simulink model "Quad_Nonlinear_LQDG"  (R2020a)
settings: Solver=ode4  StartTime=0.0  StopTime=1  FixedStep=0.02  RelTol=1e-3
InitFcn:
  | init
undefined symbols (not defined in the file or in its folder): A1, A2, A3, A4, A5, B1, B2, B3, B4, B5, C1, C2, C3, magnitude, rad, s, weighting_matrix, x0
libraries: aerolibconvert2 x4
settings Model: Creator=Ali  LastModifiedBy=Ali
settings SolverCC: AlgebraicLoopSolver=LineSearch

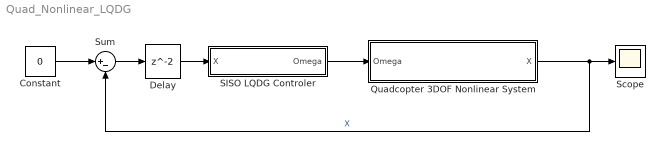
== system Quad_Nonlinear_LQDG ==
  Constant : Constant  Value=0
  Delay : Delay
  Quadcopter 3DOF Nonlinear System : Subsystem  TreatAsAtomicUnit=on
  SISO LQDG Controler : Subsystem
  Scope : Scope
  Sum : Sum  Inputs=|+-
  wires:
  Quadcopter 3DOF Nonlinear System/1(X) -> Sum/2, Scope/1  "X"
  Sum/1 -> Delay/1
  Constant/1 -> Sum/1
  Delay/1 -> SISO LQDG Controler/1(X)
  SISO LQDG Controler/1(Omega) -> Quadcopter 3DOF Nonlinear System/1(Omega)

== system Quad_Nonlinear_LQDG/Quadcopter 3DOF Nonlinear System ==
  Omega : Inport
  Integrator : Integrator  InitialCondition=x0
  Quad System : Subsystem
  Subsystem : Subsystem
  X : Outport
  wires:
  Integrator/1 -> Quad System/1(X), X/1  "X"
  Quad System/1(dot(X)) -> Integrator/1  "dot(X)"
  Omega/1 -> Subsystem/1(motor command)
  Subsystem/1(motor output) -> Quad System/2(Omega)

== system Quad_Nonlinear_LQDG/SISO LQDG Controler ==
  X : Inport
  Angular Velocity Conversion : aerolibconvert2/Angular Velocity Conversion  IU=rad/s  OU=rpm
  Angular Velocity Conversion1 : aerolibconvert2/Angular Velocity Conversion  IU=rpm  OU=rad/s
  SISO LQDG : Subsystem
  Saturation : Saturate  UpperLimit=6000  LowerLimit=1300
  u2Omega : Subsystem
  Omega : Outport
  wires:
  X/1 -> SISO LQDG/1(X)
  SISO LQDG/1(u) -> u2Omega/1(u)
  Angular Velocity Conversion/1 -> Saturation/1
  Saturation/1 -> Angular Velocity Conversion1/1
  u2Omega/1(Omega) -> Angular Velocity Conversion/1
  Angular Velocity Conversion1/1 -> Omega/1

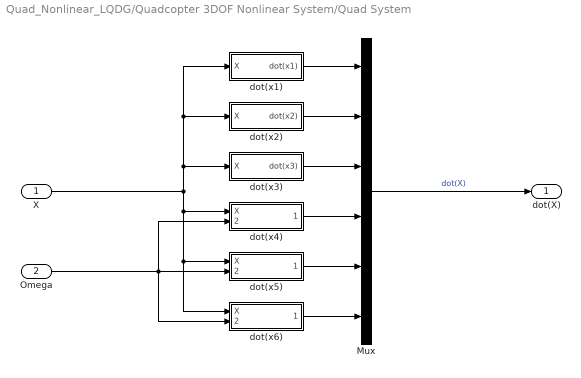
== system Quad_Nonlinear_LQDG/Quadcopter 3DOF Nonlinear System/Quad System ==
  X : Inport
  Omega : Inport  Port=2
  Mux : Mux  Inputs=6
  dot(x1) : Subsystem
  dot(x2) : Subsystem
  dot(x3) : Subsystem
  dot(x4) : Subsystem
  dot(x5) : Subsystem
  dot(x6) : Subsystem
  dot(X) : Outport
  wires:
  Mux/1 -> dot(X)/1  "dot(X)"
  X/1 -> dot(x1)/1(X), dot(x2)/1(X), dot(x3)/1(X), dot(x6)/1(X), dot(x5)/1(X), dot(x4)/1(X)
  Omega/1 -> dot(x4)/2(Omega), dot(x6)/2(Omega), dot(x5)/2(Omega)
  dot(x5)/1(dot(x5)) -> Mux/5
  dot(x2)/1(dot(x2)) -> Mux/2
  dot(x4)/1(dot(x4)) -> Mux/4
  dot(x3)/1(dot(x3)) -> Mux/3
  dot(x1)/1(dot(x1)) -> Mux/1
  dot(x6)/1(dot(x6)) -> Mux/6

== system Quad_Nonlinear_LQDG/Quadcopter 3DOF Nonlinear System/Subsystem ==
  motor command : Inport
  Angular Velocity Conversion : aerolibconvert2/Angular Velocity Conversion  IU=rad/s  OU=rpm
  Angular Velocity Conversion1 : aerolibconvert2/Angular Velocity Conversion  IU=rpm  OU=rad/s
  Mototr Transfer function : Subsystem
  Saturation : Saturate  UpperLimit=6000  LowerLimit=1300
  duty2rpm_Emax1 : Lookup_n-D  NumberOfTableDimensions=1  BreakpointsForDimension1=|  Table=|  RndMeth=Simplest  InputSameDT=on
      BreakpointsForDimension1=|
      | [0.5
      | 0.55
      | 0.6
      | 0.65
      | 0.7
      | 0.75
      | 0.8
      | 0.85
      | 0.9
      | 0.95
      | 1]
      Table=|
      | [1201
      | 2305
      | 3096
      | 3930
      | 4118
      | 4555
      | 5122
      | 5552
      | 5957
      | 6291
      | 6360]
  rpm2duty_Emax : Lookup_n-D  NumberOfTableDimensions=1  BreakpointsForDimension1=|  Table=|  RndMeth=Simplest  InputSameDT=on
      BreakpointsForDimension1=|
      | [1201
      | 2305
      | 3096
      | 3930
      | 4118
      | 4555
      | 5122
      | 5552
      | 5957
      | 6291
      | 6360]
      Table=|
      | [0.5
      | 0.55
      | 0.6
      | 0.65
      | 0.7
      | 0.75
      | 0.8
      | 0.85
      | 0.9
      | 0.95
      | 1]
  motor output : Outport
  wires:
  motor command/1 -> Angular Velocity Conversion/1
  Saturation/1 -> rpm2duty_Emax/1
  Angular Velocity Conversion/1 -> Saturation/1
  duty2rpm_Emax1/1 -> Angular Velocity Conversion1/1
  Angular Velocity Conversion1/1 -> motor output/1
  rpm2duty_Emax/1 -> Mototr Transfer function/1(In1)
  Mototr Transfer function/1(Out1) -> duty2rpm_Emax1/1

== system Quad_Nonlinear_LQDG/SISO LQDG Controler/SISO LQDG ==
  X : Inport
  Mux : Mux  Inputs=3
  Pitch LQDG Controller : Subsystem
  Roll LQDG Controller : Subsystem
  Subsystem : Subsystem
  Yaw LQDG Controller : Subsystem
  u : Outport
  wires:
  Mux/1 -> u/1  "u"
  X/1 -> Subsystem/1(X)
  Subsystem/1(roll) -> Roll LQDG Controller/1(roll)
  Roll LQDG Controller/1(u1) -> Mux/1
  Subsystem/2(pitch) -> Pitch LQDG Controller/1(pitch)
  Pitch LQDG Controller/1(u2) -> Mux/2
  Subsystem/3(yaw) -> Yaw LQDG Controller/1(yaw)
  Yaw LQDG Controller/1(u3) -> Mux/3

== system Quad_Nonlinear_LQDG/SISO LQDG Controler/u2Omega ==
  u : Inport
  MATLAB Function1 : MATLAB Function  TreatAsAtomicUnit=on
  Mux1 : Mux
  Omega : Outport
  wires:
  Mux1/1 -> Omega/1
  MATLAB Function1/2(omega_2) -> Mux1/2
  u/1 -> MATLAB Function1/1(u)
  MATLAB Function1/3(omega_3) -> Mux1/3
  MATLAB Function1/1(omega_1) -> Mux1/1
  MATLAB Function1/4(omega_4) -> Mux1/4

== system Quad_Nonlinear_LQDG/Quadcopter 3DOF Nonlinear System/Quad System/dot(x1) ==
  X : Inport
  1 : Subsystem
  Add : Sum  Inputs=+++
  Subsystem : Subsystem
  Subsystem1 : Subsystem
  dot(x1) : Outport
  wires:
  X/1 -> Subsystem1/1(X), Subsystem/1(X), 1/1(X)  "X"
  Subsystem1/1(x4) -> Add/3
  Subsystem/1(x6cos(x1)tan(x2)) -> Add/2
  Add/1 -> dot(x1)/1
  1/1(x5sin(x1)tan(x2)) -> Add/1

== system Quad_Nonlinear_LQDG/Quadcopter 3DOF Nonlinear System/Quad System/dot(x2) ==
  X : Inport
  1 : Subsystem
  Add : Sum  Inputs=+-
  Subsystem : Subsystem
  dot(x2) : Outport
  wires:
  X/1 -> 1/1(X), Subsystem/1(X)  "X"
  Subsystem/1(x6sin(x1)) -> Add/2
  Add/1 -> dot(x2)/1
  1/1(x5cos(x1)) -> Add/1

== system Quad_Nonlinear_LQDG/Quadcopter 3DOF Nonlinear System/Quad System/dot(x3) ==
  X : Inport
  1 : Subsystem
  Add : Sum
  Product : Product
  Subsystem : Subsystem
  Subsystem1 : Subsystem
  dot(x3) : Outport
  wires:
  X/1 -> Subsystem1/1(X), Subsystem/1(X), 1/1(X)  "X"
  Subsystem/1(x6cos(x1)) -> Add/2
  1/1(x5sin(x1)) -> Add/1
  Product/1 -> dot(x3)/1
  Add/1 -> Product/1
  Subsystem1/1(sec(x2)) -> Product/2

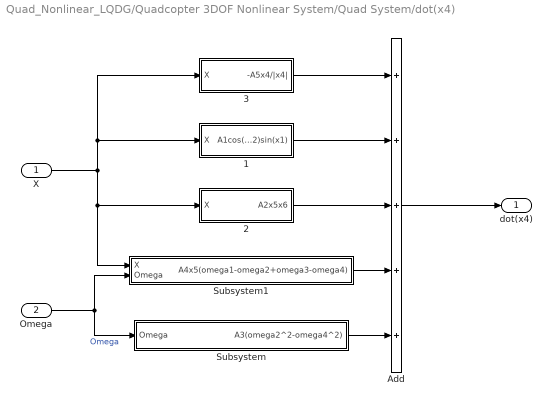
== system Quad_Nonlinear_LQDG/Quadcopter 3DOF Nonlinear System/Quad System/dot(x4) ==
  X : Inport
  Omega : Inport  Port=2
  1 : Subsystem
  2 : Subsystem
  3 : Subsystem
  Add : Sum  Inputs=+++++
  Subsystem : Subsystem
  Subsystem1 : Subsystem
  dot(x4) : Outport
  wires:
  X/1 -> Subsystem1/1(X), 2/1(X), 3/1(X), 1/1(X)
  Omega/1 -> Subsystem1/2(Omega), Subsystem/1(Omega)  "Omega"
  Add/1 -> dot(x4)/1
  3/1("-A5x4/|x4| ") -> Add/1
  1/1(A1cos(x2)sin(x1)) -> Add/2
  2/1(A2x5x6) -> Add/3
  Subsystem1/1(A4x5(omega1-omega2+omega3-omega4)) -> Add/4
  Subsystem/1(A3(omega2^2-omega4^2)) -> Add/5

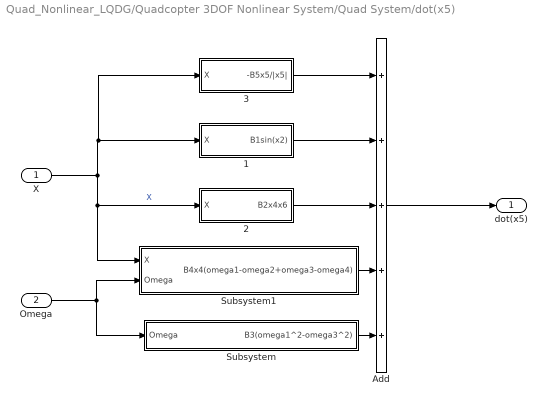
== system Quad_Nonlinear_LQDG/Quadcopter 3DOF Nonlinear System/Quad System/dot(x5) ==
  X : Inport
  Omega : Inport  Port=2
  1 : Subsystem
  2 : Subsystem
  3 : Subsystem
  Add : Sum  Inputs=+++++
  Subsystem : Subsystem
  Subsystem1 : Subsystem
  dot(x5) : Outport
  wires:
  X/1 -> Subsystem1/1(X), 2/1(X), 3/1(X), 1/1(X)  "X"
  Omega/1 -> Subsystem/1(Omega), Subsystem1/2(Omega)
  Add/1 -> dot(x5)/1
  3/1("-B5x5/|x5| ") -> Add/1
  1/1(B1sin(x2)) -> Add/2
  2/1(B2x4x6) -> Add/3
  Subsystem1/1(B4x4(omega1-omega2+omega3-omega4)) -> Add/4
  Subsystem/1(B3(omega1^2-omega3^2)) -> Add/5

== system Quad_Nonlinear_LQDG/Quadcopter 3DOF Nonlinear System/Quad System/dot(x6) ==
  X : Inport
  Omega : Inport  Port=2
  2 : Subsystem
  3 : Subsystem
  Add : Sum  Inputs=+++
  Subsystem : Subsystem
  dot(x6) : Outport
  wires:
  Omega/1 -> Subsystem/1(Omega)  "Omega"
  Add/1 -> dot(x6)/1
  3/1("-C3x6/|x6| ") -> Add/1
  2/1(C1x4x5) -> Add/2
  Subsystem/1(C2(omega1^2-omega2^2+omega3^2-omega4^2)) -> Add/3
  X/1 -> 3/1(X), 2/1(X)  "X"

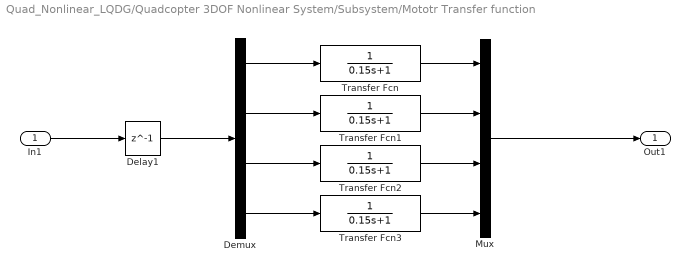
== system Quad_Nonlinear_LQDG/Quadcopter 3DOF Nonlinear System/Subsystem/Mototr Transfer function ==
  In1 : Inport
  Delay1 : Delay  DelayLength=1
  Demux : Demux
  Mux : Mux
  Transfer Fcn{,1..3} (4 alike) : TransferFcn  Denominator=[0.15 1]
  Out1 : Outport
  wires:
  Mux/1 -> Out1/1
  Transfer Fcn/1 -> Mux/1
  Delay1/1 -> Demux/1
  Demux/1 -> Transfer Fcn/1
  Transfer Fcn1/1 -> Mux/2
  Demux/3 -> Transfer Fcn2/1
  In1/1 -> Delay1/1
  Demux/2 -> Transfer Fcn1/1
  Transfer Fcn3/1 -> Mux/4
  Transfer Fcn2/1 -> Mux/3
  Demux/4 -> Transfer Fcn3/1

== system Quad_Nonlinear_LQDG/SISO LQDG Controler/SISO LQDG/Pitch LQDG Controller ==
  pitch : Inport
  Constant : Constant  Value=B1
  Constant1 : Constant  Value=B3
  Demux : Demux  Outputs=3
  Pitch function : MATLAB Function  TreatAsAtomicUnit=on
  Selector : Selector  InputPortWidth=5  IndexOptions=Index vector (dialog)  Indices=[1 3 5]  OutputSizes=1
  weighting matrix for distubance and noise using TCACS : Constant  Value=weighting_matrix
  u2 : Outport
  wires:
  Pitch function/1(u2) -> u2/1
  Demux/1 -> Pitch function/2(q_pitch)
  Demux/3 -> Pitch function/4(R_weight)
  Selector/1 -> Demux/1
  Demux/2 -> Pitch function/3(q_q)
  weighting matrix for distubance and noise using TCACS/1 -> Selector/1
  pitch/1 -> Pitch function/1(pitch)
  Constant/1 -> Pitch function/5(B1)
  Constant1/1 -> Pitch function/6(B3)

== system Quad_Nonlinear_LQDG/SISO LQDG Controler/SISO LQDG/Roll LQDG Controller ==
  roll : Inport
  Constant : Constant  Value=A1
  Constant1 : Constant  Value=A3
  Demux : Demux  Outputs=3
  Roll Function : MATLAB Function  TreatAsAtomicUnit=on
  Selector : Selector  InputPortWidth=5  IndexOptions=Index vector (dialog)  Indices=[1 3 5]  OutputSizes=1
  weighting matrix for distubance and noise using TCACS : Constant  Value=weighting_matrix
  u1 : Outport
  wires:
  Roll Function/1(u1) -> u1/1
  roll/1 -> Roll Function/1(roll)
  Demux/1 -> Roll Function/2(q_roll)
  Demux/2 -> Roll Function/3(q_p)
  Demux/3 -> Roll Function/4(R_weight)
  Selector/1 -> Demux/1
  weighting matrix for distubance and noise using TCACS/1 -> Selector/1
  Constant/1 -> Roll Function/5(A1)
  Constant1/1 -> Roll Function/6(A3)

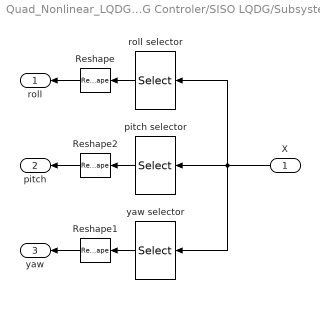
== system Quad_Nonlinear_LQDG/SISO LQDG Controler/SISO LQDG/Subsystem ==
  X : Inport
  Reshape : Reshape  OutputDimensionality=Column vector (2-D)
  Reshape1 : Reshape  OutputDimensionality=Column vector (2-D)
  Reshape2 : Reshape  OutputDimensionality=Column vector (2-D)
  pitch selector : Selector  InputPortWidth=6  IndexOptions=Index vector (dialog)  Indices=[2 5]  OutputSizes=1
  roll selector : Selector  InputPortWidth=6  IndexOptions=Index vector (dialog)  Indices=[1 4]  OutputSizes=1
  yaw selector : Selector  InputPortWidth=6  IndexOptions=Index vector (dialog)  Indices=[3 6]  OutputSizes=1
  roll : Outport
  pitch : Outport  Port=2
  yaw : Outport  Port=3
  wires:
  X/1 -> yaw selector/1, roll selector/1, pitch selector/1
  roll selector/1 -> Reshape/1
  pitch selector/1 -> Reshape2/1
  yaw selector/1 -> Reshape1/1
  Reshape/1 -> roll/1
  Reshape2/1 -> pitch/1
  Reshape1/1 -> yaw/1

== system Quad_Nonlinear_LQDG/SISO LQDG Controler/SISO LQDG/Yaw LQDG Controller ==
  yaw : Inport
  Constant : Constant  Value=C2
  Demux : Demux  Outputs=3
  Selector : Selector  InputPortWidth=5  IndexOptions=Index vector (dialog)  Indices=[2 4 5]  OutputSizes=1
  Yaw function : MATLAB Function  TreatAsAtomicUnit=on
  weighting matrix using TCACS : Constant  Value=weighting_matrix
  u3 : Outport
  wires:
  Demux/2 -> Yaw function/3(q_r)
  Demux/1 -> Yaw function/2(q_yaw)
  Yaw function/1(u3) -> u3/1
  Demux/3 -> Yaw function/4(R_weight)
  yaw/1 -> Yaw function/1(yaw)
  weighting matrix using TCACS/1 -> Selector/1
  Selector/1 -> Demux/1
  Constant/1 -> Yaw function/5(C2)

== system Quad_Nonlinear_LQDG/Quadcopter 3DOF Nonlinear System/Quad System/dot(x1)/1 ==
  X : Inport
  Demux : Demux  Outputs=6
  Subsystem : Subsystem
  Terminator : Terminator
  Terminator1 : Terminator
  Terminator2 : Terminator
  x5sin(x1)tan(x2) : Outport
  wires:
  Demux/2 -> Subsystem/2(x2)  "x2"
  Demux/4 -> Terminator1/1  "x4"
  X/1 -> Demux/1  "x"
  Demux/1 -> Subsystem/1(x1)  "x1"
  Demux/3 -> Terminator/1  "x3"
  Demux/6 -> Terminator2/1  "x6"
  Demux/5 -> Subsystem/3(x5)  "x5"
  Subsystem/1(x5sin(x1)tan(x2)) -> x5sin(x1)tan(x2)/1

== system Quad_Nonlinear_LQDG/Quadcopter 3DOF Nonlinear System/Quad System/dot(x1)/Subsystem ==
  X : Inport
  Demux : Demux  Outputs=6
  Subsystem1 : Subsystem
  Terminator : Terminator
  Terminator1 : Terminator
  Terminator3 : Terminator
  x6cos(x1)tan(x2) : Outport
  wires:
  Demux/1 -> Subsystem1/1(x1)  "x1"
  Demux/3 -> Terminator/1  "x3"
  Demux/4 -> Terminator1/1  "x4"
  Demux/5 -> Terminator3/1  "x5"
  Demux/6 -> Subsystem1/3(x6)  "x6"
  Subsystem1/1(x6cos(x1)tan(x2)) -> x6cos(x1)tan(x2)/1  "x6cos(x1)tan(x2)"
  X/1 -> Demux/1  "X"
  Demux/2 -> Subsystem1/2(x2)  "x2"

== system Quad_Nonlinear_LQDG/Quadcopter 3DOF Nonlinear System/Quad System/dot(x1)/Subsystem1 ==
  X : Inport
  Demux : Demux  Outputs=6
  Terminator{,2..5} (5 alike) : Terminator
  x4 : Outport
  wires:
  Demux/6 -> Terminator5/1  "x6"
  X/1 -> Demux/1
  Demux/3 -> Terminator/1  "x3"
  Demux/1 -> Terminator4/1  "x1"
  Demux/2 -> Terminator2/1  "x2"
  Demux/5 -> Terminator3/1  "x5"
  Demux/4 -> x4/1  "x4"

== system Quad_Nonlinear_LQDG/Quadcopter 3DOF Nonlinear System/Quad System/dot(x2)/1 ==
  X : Inport
  Demux : Demux  Outputs=6
  Subsystem : Subsystem
  Terminator{,1..3} (4 alike) : Terminator
  x5cos(x1) : Outport
  wires:
  Demux/4 -> Terminator1/1  "x4"
  X/1 -> Demux/1  "x"
  Demux/1 -> Subsystem/1(x1)  "x1"
  Demux/3 -> Terminator/1  "x3"
  Demux/6 -> Terminator2/1  "x6"
  Demux/5 -> Subsystem/2(x5)  "x5"
  Subsystem/1(Out1) -> x5cos(x1)/1
  Demux/2 -> Terminator3/1  "x2"

== system Quad_Nonlinear_LQDG/Quadcopter 3DOF Nonlinear System/Quad System/dot(x2)/Subsystem ==
  X : Inport
  Demux : Demux  Outputs=6
  Subsystem1 : Subsystem
  Terminator{,1..3} (4 alike) : Terminator
  x6sin(x1) : Outport
  wires:
  Demux/1 -> Subsystem1/1(x1)  "x1"
  Demux/3 -> Terminator/1  "x3"
  Demux/4 -> Terminator1/1  "x4"
  Demux/5 -> Terminator3/1  "x5"
  Demux/6 -> Subsystem1/2(x6)  "x6"
  Subsystem1/1(Out1) -> x6sin(x1)/1  "x6sin(x1)"
  X/1 -> Demux/1  "X"
  Demux/2 -> Terminator2/1  "x2"

== system Quad_Nonlinear_LQDG/Quadcopter 3DOF Nonlinear System/Quad System/dot(x3)/1 ==
  X : Inport
  Demux : Demux  Outputs=6
  Subsystem : Subsystem
  Terminator{,1..3} (4 alike) : Terminator
  x5sin(x1) : Outport
  wires:
  Demux/4 -> Terminator1/1  "x4"
  X/1 -> Demux/1  "x"
  Demux/1 -> Subsystem/1(x1)  "x1"
  Demux/3 -> Terminator/1  "x3"
  Demux/6 -> Terminator2/1  "x6"
  Demux/5 -> Subsystem/2(x5)  "x5"
  Subsystem/1(x5sin(x1)) -> x5sin(x1)/1
  Demux/2 -> Terminator3/1  "x2"

== system Quad_Nonlinear_LQDG/Quadcopter 3DOF Nonlinear System/Quad System/dot(x3)/Subsystem ==
  X : Inport
  Demux : Demux  Outputs=6
  Subsystem1 : Subsystem
  Terminator{,1..3} (4 alike) : Terminator
  x6cos(x1) : Outport
  wires:
  Demux/1 -> Subsystem1/1(x1)  "x1"
  Demux/3 -> Terminator/1  "x3"
  Demux/4 -> Terminator1/1  "x4"
  Demux/5 -> Terminator3/1  "x5"
  Demux/6 -> Subsystem1/2(x6)  "x6"
  Subsystem1/1(Out1) -> x6cos(x1)/1  "x6cos(x1)"
  X/1 -> Demux/1  "X"
  Demux/2 -> Terminator2/1  "x2"

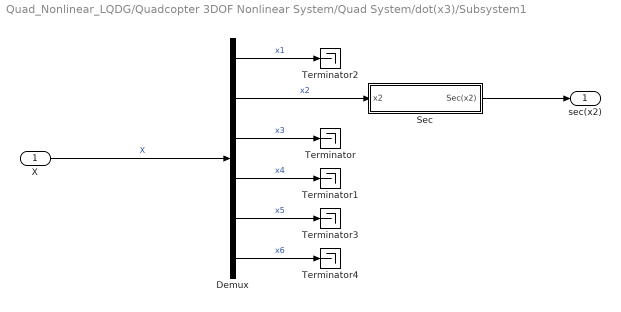
== system Quad_Nonlinear_LQDG/Quadcopter 3DOF Nonlinear System/Quad System/dot(x3)/Subsystem1 ==
  X : Inport
  Demux : Demux  Outputs=6
  Sec : Subsystem
  Terminator{,1..4} (5 alike) : Terminator
  sec(x2) : Outport
  wires:
  Demux/3 -> Terminator/1  "x3"
  Demux/4 -> Terminator1/1  "x4"
  Demux/5 -> Terminator3/1  "x5"
  X/1 -> Demux/1  "X"
  Demux/1 -> Terminator2/1  "x1"
  Demux/6 -> Terminator4/1  "x6"
  Demux/2 -> Sec/1(x2)  "x2"
  Sec/1(Sec(x2)) -> sec(x2)/1

== system Quad_Nonlinear_LQDG/Quadcopter 3DOF Nonlinear System/Quad System/dot(x4)/1 ==
  X : Inport
  Demux : Demux  Outputs=6
  Subsystem : Subsystem
  Terminator{,1..3} (4 alike) : Terminator
  A1cos(x2)sin(x1) : Outport
  wires:
  Demux/4 -> Terminator1/1  "x4"
  X/1 -> Demux/1  "x"
  Demux/1 -> Subsystem/1(x1)  "x1"
  Demux/3 -> Terminator/1  "x3"
  Demux/6 -> Terminator2/1  "x6"
  Subsystem/1(A1cos(x2)sin(x1)) -> A1cos(x2)sin(x1)/1
  Demux/2 -> Subsystem/2(x2)  "x2"
  Demux/5 -> Terminator3/1  "x5"

== system Quad_Nonlinear_LQDG/Quadcopter 3DOF Nonlinear System/Quad System/dot(x4)/2 ==
  X : Inport
  Demux : Demux  Outputs=6
  Subsystem : Subsystem
  Terminator{,1,4..5} (4 alike) : Terminator
  A2x5x6 : Outport
  wires:
  Demux/4 -> Terminator1/1  "x4"
  X/1 -> Demux/1  "x"
  Demux/3 -> Terminator/1  "x3"
  Demux/6 -> Subsystem/2(x6)  "x6"
  Subsystem/1(A2x5x6) -> A2x5x6/1
  Demux/5 -> Subsystem/1(x5)  "x5"
  Demux/1 -> Terminator4/1  "x1"
  Demux/2 -> Terminator5/1  "x2"

== system Quad_Nonlinear_LQDG/Quadcopter 3DOF Nonlinear System/Quad System/dot(x4)/3 ==
  X : Inport
  Demux : Demux  Outputs=6
  Subsystem : Subsystem
  Terminator{,2..5} (5 alike) : Terminator
  "-A5x4/|x4| " : Outport
  wires:
  X/1 -> Demux/1  "x"
  Demux/1 -> Terminator5/1  "x1"
  Demux/3 -> Terminator/1  "x3"
  Demux/6 -> Terminator2/1  "x6"
  Demux/2 -> Terminator4/1  "x2"
  Demux/5 -> Terminator3/1  "x5"
  Demux/4 -> Subsystem/1(x4)  "x4"
  Subsystem/1("-A5x4/|x4| ") -> "-A5x4/|x4| "/1

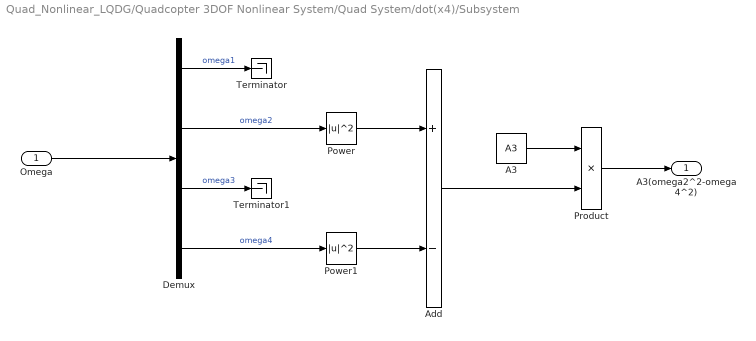
== system Quad_Nonlinear_LQDG/Quadcopter 3DOF Nonlinear System/Quad System/dot(x4)/Subsystem ==
  Omega : Inport
  A3 : Constant  Value=A3
  Add : Sum  Inputs=+-
  Demux : Demux
  Power : Math  Operator=magnitude^2  SaturateOnIntegerOverflow=on
  Power1 : Math  Operator=magnitude^2  SaturateOnIntegerOverflow=on
  Product : Product
  Terminator : Terminator
  Terminator1 : Terminator
  A3(omega2^2-omega4^2) : Outport
  wires:
  Product/1 -> A3(omega2^2-omega4^2)/1
  Power1/1 -> Add/2
  Demux/2 -> Power/1  "omega2"
  Demux/4 -> Power1/1  "omega4"
  Add/1 -> Product/2
  Power/1 -> Add/1
  A3/1 -> Product/1
  Omega/1 -> Demux/1
  Demux/3 -> Terminator1/1  "omega3"
  Demux/1 -> Terminator/1  "omega1"

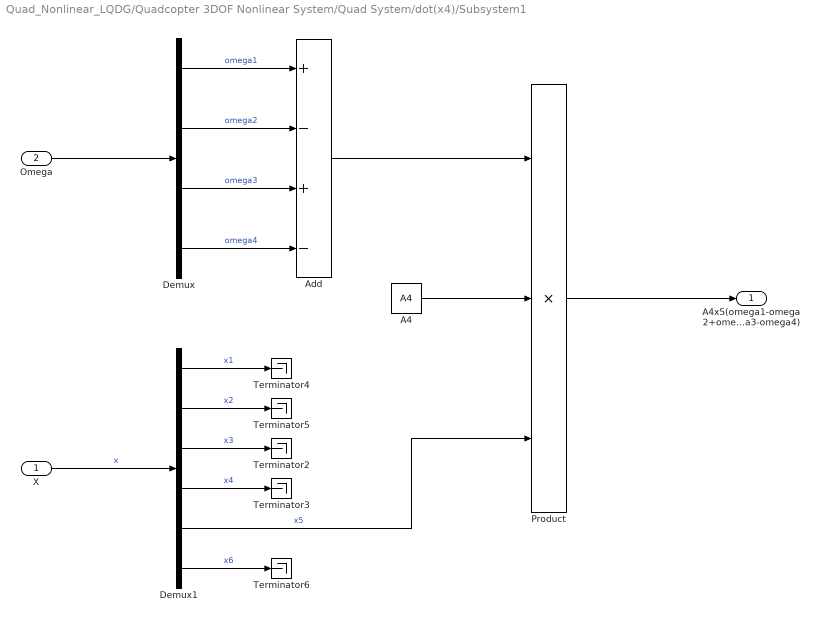
== system Quad_Nonlinear_LQDG/Quadcopter 3DOF Nonlinear System/Quad System/dot(x4)/Subsystem1 ==
  X : Inport
  Omega : Inport  Port=2
  A4 : Constant  Value=A4
  Add : Sum  Inputs=+-+-
  Demux : Demux
  Demux1 : Demux  Outputs=6
  Product : Product  Inputs=3
  Terminator{2..6} (5 alike) : Terminator
  A4x5(omega1-omega2+omega3-omega4) : Outport
  wires:
  Omega/1 -> Demux/1
  Demux1/6 -> Terminator6/1  "x6"
  Demux1/5 -> Product/3  "x5"
  X/1 -> Demux1/1  "x"
  Demux1/2 -> Terminator5/1  "x2"
  Demux1/3 -> Terminator2/1  "x3"
  Demux1/4 -> Terminator3/1  "x4"
  Demux1/1 -> Terminator4/1  "x1"
  Demux/1 -> Add/1  "omega1"
  Demux/2 -> Add/2  "omega2"
  Demux/3 -> Add/3  "omega3"
  Demux/4 -> Add/4  "omega4"
  Add/1 -> Product/1
  A4/1 -> Product/2
  Product/1 -> A4x5(omega1-omega2+omega3-omega4)/1

== system Quad_Nonlinear_LQDG/Quadcopter 3DOF Nonlinear System/Quad System/dot(x5)/1 ==
  X : Inport
  Demux : Demux  Outputs=6
  Subsystem : Subsystem
  Terminator{,1..4} (5 alike) : Terminator
  B1sin(x2) : Outport
  wires:
  Demux/4 -> Terminator1/1  "x4"
  X/1 -> Demux/1  "x"
  Demux/3 -> Terminator/1  "x3"
  Demux/6 -> Terminator2/1  "x6"
  Subsystem/1(B1sin(x2)) -> B1sin(x2)/1
  Demux/2 -> Subsystem/1(x2)  "x2"
  Demux/5 -> Terminator3/1  "x5"
  Demux/1 -> Terminator4/1  "x1"

== system Quad_Nonlinear_LQDG/Quadcopter 3DOF Nonlinear System/Quad System/dot(x5)/2 ==
  X : Inport
  Demux : Demux  Outputs=6
  Subsystem : Subsystem
  Terminator{,2,4..5} (4 alike) : Terminator
  B2x4x6 : Outport
  wires:
  Demux/4 -> Subsystem/1(x4)  "x4"
  X/1 -> Demux/1  "x"
  Demux/3 -> Terminator/1  "x3"
  Demux/6 -> Subsystem/2(x6)  "x6"
  Subsystem/1(B2x4x6) -> B2x4x6/1
  Demux/1 -> Terminator4/1  "x1"
  Demux/2 -> Terminator5/1  "x2"
  Demux/5 -> Terminator2/1  "x5"

== system Quad_Nonlinear_LQDG/Quadcopter 3DOF Nonlinear System/Quad System/dot(x5)/3 ==
  X : Inport
  Demux : Demux  Outputs=6
  Subsystem : Subsystem
  Terminator{,1..2,4..5} (5 alike) : Terminator
  "-B5x5/|x5| " : Outport
  wires:
  X/1 -> Demux/1  "x"
  Demux/1 -> Terminator5/1  "x1"
  Demux/3 -> Terminator/1  "x3"
  Demux/6 -> Terminator2/1  "x6"
  Demux/2 -> Terminator4/1  "x2"
  Demux/5 -> Subsystem/1(x5)  "x5"
  Subsystem/1("-B5x5/|x5| ") -> "-B5x5/|x5| "/1
  Demux/4 -> Terminator1/1  "x4"

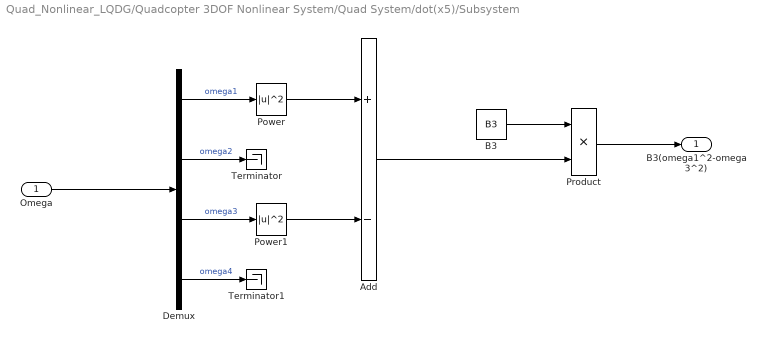
== system Quad_Nonlinear_LQDG/Quadcopter 3DOF Nonlinear System/Quad System/dot(x5)/Subsystem ==
  Omega : Inport
  Add : Sum  Inputs=+-
  B3 : Constant  Value=B3
  Demux : Demux
  Power : Math  Operator=magnitude^2  SaturateOnIntegerOverflow=on
  Power1 : Math  Operator=magnitude^2  SaturateOnIntegerOverflow=on
  Product : Product
  Terminator : Terminator
  Terminator1 : Terminator
  B3(omega1^2-omega3^2) : Outport
  wires:
  Product/1 -> B3(omega1^2-omega3^2)/1
  Power1/1 -> Add/2
  Add/1 -> Product/2
  Power/1 -> Add/1
  B3/1 -> Product/1
  Omega/1 -> Demux/1
  Demux/3 -> Power1/1  "omega3"
  Demux/1 -> Power/1  "omega1"
  Demux/2 -> Terminator/1  "omega2"
  Demux/4 -> Terminator1/1  "omega4"

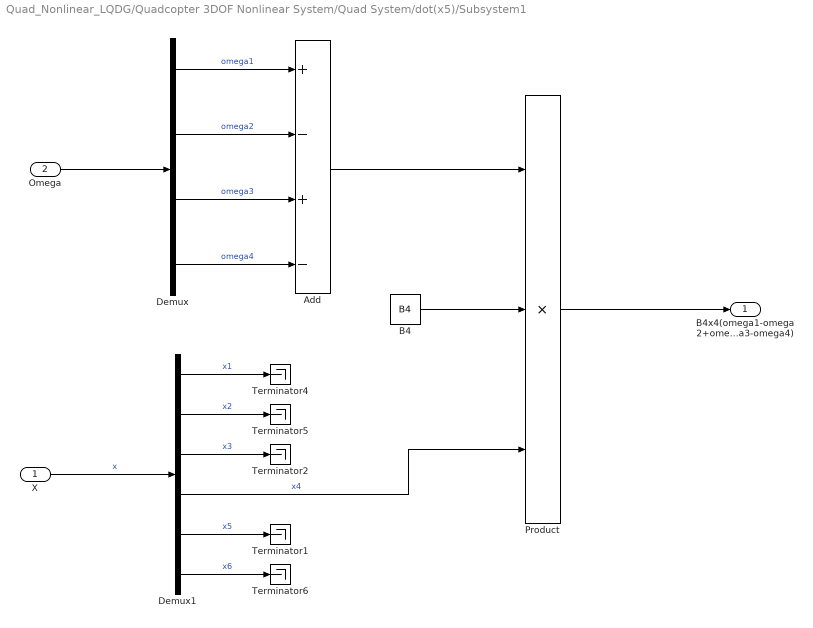
== system Quad_Nonlinear_LQDG/Quadcopter 3DOF Nonlinear System/Quad System/dot(x5)/Subsystem1 ==
  X : Inport
  Omega : Inport  Port=2
  Add : Sum  Inputs=+-+-
  B4 : Constant  Value=B4
  Demux : Demux
  Demux1 : Demux  Outputs=6
  Product : Product  Inputs=3
  Terminator{1..2,4..6} (5 alike) : Terminator
  B4x4(omega1-omega2+omega3-omega4) : Outport
  wires:
  Omega/1 -> Demux/1
  Demux1/6 -> Terminator6/1  "x6"
  X/1 -> Demux1/1  "x"
  Demux1/2 -> Terminator5/1  "x2"
  Demux1/3 -> Terminator2/1  "x3"
  Demux1/4 -> Product/3  "x4"
  Demux1/1 -> Terminator4/1  "x1"
  Demux/1 -> Add/1  "omega1"
  Demux/2 -> Add/2  "omega2"
  Demux/3 -> Add/3  "omega3"
  Demux/4 -> Add/4  "omega4"
  Add/1 -> Product/1
  B4/1 -> Product/2
  Product/1 -> B4x4(omega1-omega2+omega3-omega4)/1
  Demux1/5 -> Terminator1/1  "x5"

== system Quad_Nonlinear_LQDG/Quadcopter 3DOF Nonlinear System/Quad System/dot(x6)/2 ==
  X : Inport
  Demux : Demux  Outputs=6
  Subsystem : Subsystem
  Terminator{,2,4..5} (4 alike) : Terminator
  C1x4x5 : Outport
  wires:
  Demux/4 -> Subsystem/1(x4)  "x4"
  X/1 -> Demux/1  "x"
  Demux/3 -> Terminator/1  "x3"
  Subsystem/1(C1x4x5) -> C1x4x5/1
  Demux/1 -> Terminator4/1  "x1"
  Demux/2 -> Terminator5/1  "x2"
  Demux/5 -> Subsystem/2(x5)  "x5"
  Demux/6 -> Terminator2/1  "x6"

== system Quad_Nonlinear_LQDG/Quadcopter 3DOF Nonlinear System/Quad System/dot(x6)/3 ==
  X : Inport
  Demux : Demux  Outputs=6
  Subsystem : Subsystem
  Terminator{,1,3..5} (5 alike) : Terminator
  "-C3x6/|x6| " : Outport
  wires:
  X/1 -> Demux/1  "x"
  Demux/1 -> Terminator5/1  "x1"
  Demux/3 -> Terminator/1  "x3"
  Demux/6 -> Subsystem/1(x6)  "x6"
  Demux/2 -> Terminator4/1  "x2"
  Demux/5 -> Terminator3/1  "x5"
  Subsystem/1("-C3x6/|x6| ") -> "-C3x6/|x6| "/1
  Demux/4 -> Terminator1/1  "x4"

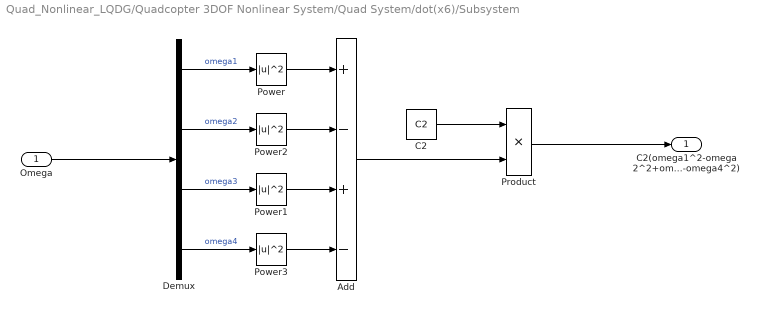
== system Quad_Nonlinear_LQDG/Quadcopter 3DOF Nonlinear System/Quad System/dot(x6)/Subsystem ==
  Omega : Inport
  Add : Sum  Inputs=+-+-
  C2 : Constant  Value=C2
  Demux : Demux
  Power{,1..3} (4 alike) : Math  Operator=magnitude^2  SaturateOnIntegerOverflow=on
  Product : Product
  C2(omega1^2-omega2^2+omega3^2-omega4^2) : Outport
  wires:
  Omega/1 -> Demux/1
  Demux/3 -> Power1/1  "omega3"
  Demux/1 -> Power/1  "omega1"
  Demux/2 -> Power2/1  "omega2"
  Demux/4 -> Power3/1  "omega4"
  C2/1 -> Product/1
  Add/1 -> Product/2
  Product/1 -> C2(omega1^2-omega2^2+omega3^2-omega4^2)/1
  Power/1 -> Add/1
  Power2/1 -> Add/2
  Power1/1 -> Add/3
  Power3/1 -> Add/4

== system Quad_Nonlinear_LQDG/Quadcopter 3DOF Nonlinear System/Quad System/dot(x1)/1/Subsystem ==
  x1 : Inport
  x2 : Inport  Port=2
  x5 : Inport  Port=3
  Product : Product  Inputs=3
  Sin : Trigonometry
  Tan : Trigonometry  Operator=tan
  x5sin(x1)tan(x2) : Outport
  wires:
  Sin/1 -> Product/1
  x5/1 -> Product/3
  Product/1 -> x5sin(x1)tan(x2)/1
  x1/1 -> Sin/1
  x2/1 -> Tan/1
  Tan/1 -> Product/2

== system Quad_Nonlinear_LQDG/Quadcopter 3DOF Nonlinear System/Quad System/dot(x1)/Subsystem/Subsystem1 ==
  x1 : Inport
  x2 : Inport  Port=2
  x6 : Inport  Port=3
  Cos : Trigonometry  Operator=cos
  Product1 : Product  Inputs=3
  Tan : Trigonometry  Operator=tan
  x6cos(x1)tan(x2) : Outport
  wires:
  x6/1 -> Product1/3
  x1/1 -> Cos/1
  Cos/1 -> Product1/1
  x2/1 -> Tan/1
  Product1/1 -> x6cos(x1)tan(x2)/1
  Tan/1 -> Product1/2

== system Quad_Nonlinear_LQDG/Quadcopter 3DOF Nonlinear System/Quad System/dot(x2)/1/Subsystem ==
  x1 : Inport
  x5 : Inport  Port=2
  Cos : Trigonometry  Operator=cos
  Product : Product
  Out1 : Outport
  wires:
  Cos/1 -> Product/1
  Product/1 -> Out1/1
  x1/1 -> Cos/1
  x5/1 -> Product/2

== system Quad_Nonlinear_LQDG/Quadcopter 3DOF Nonlinear System/Quad System/dot(x2)/Subsystem/Subsystem1 ==
  x1 : Inport
  x6 : Inport  Port=2
  Product1 : Product
  Sin : Trigonometry
  Out1 : Outport
  wires:
  x6/1 -> Product1/2
  x1/1 -> Sin/1
  Sin/1 -> Product1/1
  Product1/1 -> Out1/1

== system Quad_Nonlinear_LQDG/Quadcopter 3DOF Nonlinear System/Quad System/dot(x3)/1/Subsystem ==
  x1 : Inport
  x5 : Inport  Port=2
  Product : Product
  Sin : Trigonometry
  x5sin(x1) : Outport
  wires:
  Sin/1 -> Product/1
  Product/1 -> x5sin(x1)/1
  x1/1 -> Sin/1
  x5/1 -> Product/2

== system Quad_Nonlinear_LQDG/Quadcopter 3DOF Nonlinear System/Quad System/dot(x3)/Subsystem/Subsystem1 ==
  x1 : Inport
  x6 : Inport  Port=2
  Cos : Trigonometry  Operator=cos
  Product1 : Product
  Out1 : Outport
  wires:
  x6/1 -> Product1/2
  x1/1 -> Cos/1
  Cos/1 -> Product1/1
  Product1/1 -> Out1/1

== system Quad_Nonlinear_LQDG/Quadcopter 3DOF Nonlinear System/Quad System/dot(x3)/Subsystem1/Sec ==
  x2 : Inport
  Constant : Constant
  Cos : Trigonometry  Operator=cos
  Divide : Product  Inputs=*/
  Sec(x2) : Outport
  wires:
  Constant/1 -> Divide/1
  Cos/1 -> Divide/2
  Divide/1 -> Sec(x2)/1
  x2/1 -> Cos/1

== system Quad_Nonlinear_LQDG/Quadcopter 3DOF Nonlinear System/Quad System/dot(x4)/1/Subsystem ==
  x1 : Inport
  x2 : Inport  Port=2
  A1 : Constant  Value=A1
  Cos : Trigonometry  Operator=cos
  Product : Product  Inputs=3
  Sin : Trigonometry
  A1cos(x2)sin(x1) : Outport
  wires:
  Sin/1 -> Product/1
  Product/1 -> A1cos(x2)sin(x1)/1
  x1/1 -> Sin/1
  x2/1 -> Cos/1
  Cos/1 -> Product/2
  A1/1 -> Product/3

== system Quad_Nonlinear_LQDG/Quadcopter 3DOF Nonlinear System/Quad System/dot(x4)/2/Subsystem ==
  x5 : Inport
  x6 : Inport  Port=2
  A2 : Constant  Value=A2
  Product : Product  Inputs=3
  A2x5x6 : Outport
  wires:
  x5/1 -> Product/1
  Product/1 -> A2x5x6/1
  x6/1 -> Product/2
  A2/1 -> Product/3

== system Quad_Nonlinear_LQDG/Quadcopter 3DOF Nonlinear System/Quad System/dot(x4)/3/Subsystem ==
  x4 : Inport
  A5 : Constant  Value=A5
  Gain : Gain  Gain=-1
  Switch : Switch  Criteria=u2 > Threshold
  "-A5x4/|x4| " : Outport
  wires:
  Switch/1 -> "-A5x4/|x4| "/1
  A5/1 -> Switch/3, Gain/1
  x4/1 -> Switch/2
  Gain/1 -> Switch/1

== system Quad_Nonlinear_LQDG/Quadcopter 3DOF Nonlinear System/Quad System/dot(x5)/1/Subsystem ==
  x2 : Inport
  B1 : Constant  Value=B1
  Product : Product
  Sin : Trigonometry
  B1sin(x2) : Outport
  wires:
  Product/1 -> B1sin(x2)/1
  x2/1 -> Sin/1
  B1/1 -> Product/2
  Sin/1 -> Product/1

== system Quad_Nonlinear_LQDG/Quadcopter 3DOF Nonlinear System/Quad System/dot(x5)/2/Subsystem ==
  x4 : Inport
  x6 : Inport  Port=2
  B2 : Constant  Value=B2
  Product : Product  Inputs=3
  B2x4x6 : Outport
  wires:
  x4/1 -> Product/1
  Product/1 -> B2x4x6/1
  x6/1 -> Product/2
  B2/1 -> Product/3

== system Quad_Nonlinear_LQDG/Quadcopter 3DOF Nonlinear System/Quad System/dot(x5)/3/Subsystem ==
  x5 : Inport
  B5 : Constant  Value=B5
  Gain : Gain  Gain=-1
  Switch : Switch  Criteria=u2 > Threshold
  "-B5x5/|x5| " : Outport
  wires:
  Switch/1 -> "-B5x5/|x5| "/1
  B5/1 -> Switch/3, Gain/1
  x5/1 -> Switch/2
  Gain/1 -> Switch/1

== system Quad_Nonlinear_LQDG/Quadcopter 3DOF Nonlinear System/Quad System/dot(x6)/2/Subsystem ==
  x4 : Inport
  x5 : Inport  Port=2
  C1 : Constant  Value=C1
  Product : Product  Inputs=3
  C1x4x5 : Outport
  wires:
  x4/1 -> Product/1
  Product/1 -> C1x4x5/1
  x5/1 -> Product/2
  C1/1 -> Product/3

== system Quad_Nonlinear_LQDG/Quadcopter 3DOF Nonlinear System/Quad System/dot(x6)/3/Subsystem ==
  x6 : Inport
  C3 : Constant  Value=C3
  Gain : Gain  Gain=-1
  Switch : Switch  Criteria=u2 > Threshold
  "-C3x6/|x6| " : Outport
  wires:
  Switch/1 -> "-C3x6/|x6| "/1
  C3/1 -> Switch/3, Gain/1
  x6/1 -> Switch/2
  Gain/1 -> Switch/1

== matlab function Quad_Nonlinear_LQDG/SISO LQDG Controler/u2Omega/MATLAB Function1 ==
  data: u input size=3; omega_1 output size=1; omega_2 output size=1; omega_3 output size=1; omega_4 output size=1
function [omega_1, omega_2, omega_3, omega_4] = fcn(u)
u1 = u(1);
u2 = u(2);
u3 = u(3);
% control effort
u4 = ones(1, length(u1)) * 4 * rpm2rad_sec(2000)^2;
% calculate omega
if (u4 + u3 + 2 * u2) / 4 > 0
    omega_1 = sqrt((u4 + u3 + 2 * u2) / 4);
else
    omega_1 = 0;
end
if (u4 + u3 - 2 * u2) / 4 > 0
    omega_3 = sqrt((u4 + u3 - 2 * u2) / 4);
else
    omega_3 = 0;
end
if (u4 - u3 + 2 * u1) / 4 > 0
    omega_2 = sqrt((u4 - u3 + 2 * u1) / 4);
else
    omega_2 = 0;
end
if (u4 - u3 - 2 * u1) / 4 > 0
    omega_4 = sqrt((u4 - u3 - 2 * u1) / 4);
else
    omega_4 = 0;
end
end
%% functions
% rpm to rad/sec
function rad = rpm2rad_sec(rpm)
rad = rpm / 60 * 2 * pi;
end

== matlab function Quad_Nonlinear_LQDG/SISO LQDG Controler/SISO LQDG/Pitch LQDG Controller/Pitch function ==
  data: pitch input; u2 output; q_pitch input; q_q input; R_weight input; B1 input; B3 input
function u2 = fcn(pitch, q_pitch, q_q, R_weight, B1, B3)
% QuadConstants;
% QuadConstants;
%%% constans %%%
% Distance between rotor center to quad center (m)
% d_cg = 0.295;
% Distance between D point to quad center (m)
% h_cg = 0.0078;
% Thrust factor (non dimensional)
% b = 1.10794e-5;
% Rotor torque drag factor (non dimensional)
% d = 3.2e-6;
% Total mass (kg)
% m_tot = 1.774;
% Quad Moment of inertia respect to axix X Body (kg.m^2)
% J_xx = 0.0297598;
% Quad Moment of inertia respect to axix Y Body (kg.m^2)
% J_yy = 0.0298565;
% Quad Moment of inertia respect to axix Y Body (kg.m^2)
% J_zz = 0.058510;
% Quad blade Moment (kg.m^2)
% J_R = 4.439e-5;
% Mass on X axis bearing (kg)
% m1 = 1.272;
% Mass on Y axis bearing (kg)
% m2 = 1.074;
% Mass on Z axis bearing (kg)
% m3 = 1.693;
% Bearing radius in X axix (m)
% r_x = 0.01;
% Bearing radius in Y axix (m)
% r_y = 0.01;
% Bearing radius in Z axix (m)
% r_z = 0.025;
% Static bearing friction (non dimensional)
% miu_s = 0.003;
% Dynamic bearing friction (non dimensional)
% miu_k = 0.002;
% Motor constant (non dimensional)
% tau = 0.15;
% Delay of motor (sec)
% T_d = 0.02;
% Gravity force (m/s^2)
% g = 9.81;
% A Constants
% A1 = (h_cg * g * m_tot) / (m_tot * h_cg^2 + J_xx);
% A2 = (2*m_tot * h_cg^2 + J_yy -J_zz) / (m_tot * h_cg^2 + J_xx);
% A3 = (b * d_cg) / (m_tot * h_cg^2 + J_xx);
% A4 = (J_R) / (m_tot * h_cg^2 + J_xx);
% A5 = (m1 * g * miu_k * r_x) / (m_tot * h_cg^2 + J_xx);
% B Constants
% B1 = (h_cg * g * m_tot) / (m_tot * h_cg^2 + J_yy);
% B2 = (-2*m_tot * h_cg^2 - J_xx + J_zz) / (m_tot * h_cg^2 + J_yy);
% B3 = (b * d_cg) / (m_tot * h_cg^2 + J_yy);
% B4 = (-J_R) / (m_tot * h_cg^2 + J_yy);
% B5 = (m2 * g * miu_k * r_y) / (m_tot * h_cg^2 + J_yy);
% C Constants
% C1 = (J_xx - J_yy) / (J_zz);
% C2 = (d) / (J_zz);
% C3 = (m3 * g * miu_k * r_z) / (J_zz);
% omega for linearzation 2000 RPM
% Omega = 2000 / 60 * 2 * pi;

x2     = pitch(1);
A22    = 0; %da2dx2
A25    = 1; %da2dx5
A52    = B1 * cos(x2); %da5dx2
A55    = 0; %da5dx5

A      = [A22, A25 ;
          A52, A55];
B      = [0  ;
          B3];
a      = A(2);
b      = B(2);

q1     = 10^q_pitch;
q2     = 10^q_q;
R1     = 1;
R2     = 10^R_weight;
R1_inv = R1^-1;
R2_inv = R2^-1;
k1_ans = zeros(2, 2);
k2_ans = zeros(2, 2);

% algebraic_riccati = K * A + A' * K - K * B * R^-1 * B' * K + Q;
% first equation q1 + 2*a*k12 - (b^2*k12^2)/R = 0
% Ans1 K12 = -m*(k + (k^2 + Q11)^(1/2))
% Ans2 K12 = -m*(k - (k^2 + Q11)^(1/2))
valid_ans = false; % answer validation for statble system
k12_1 = zeros(1, 2);
k12_2 = zeros(1, 2);
k12_1(1) =   (R1*R2*a + R1*b^2*((R1*R2*(R1*R2*a^2 + R1*b^2*q1 + R2*b^2*q1))/(b^4*(R1 + R2)^2))^(1/2) + R2*b^2*((R1*R2*(R1*R2*a^2 + R1*b^2*q1 + R2*b^2*q1))/(b^4*(R1 + R2)^2))^(1/2))/(R1*b^2 + R2*b^2);
k12_1(2) =  -(R1*b^2*((R1*R2*(R1*R2*a^2 + R1*b^2*q1 + R2*b^2*q1))/(b^4*(R1 + R2)^2))^(1/2) - R1*R2*a + R2*b^2*((R1*R2*(R1*R2*a^2 + R1*b^2*q1 + R2*b^2*q1))/(b^4*(R1 + R2)^2))^(1/2))/(R1*b^2 + R2*b^2);
k12_2(1) =  (R1*R2*a + R1*b^2*((R1*R2*(R1*R2*a^2 + R1*b^2*q1 + R2*b^2*q1))/(b^4*(R1 + R2)^2))^(1/2) + R2*b^2*((R1*R2*(R1*R2*a^2 + R1*b^2*q1 + R2*b^2*q1))/(b^4*(R1 + R2)^2))^(1/2))/(R1*b^2 + R2*b^2);
for i = 1:length(k12_1)
    % Second equation 
    % 1 (b^2*k22_1^2)/R1 + (k22_2*b^2*k22_1)/R2 - 2*k12_1 - q2 = 0
    % 2 (b^2*k22_2^2)/R2 + (k22_1*b^2*k22_2)/R1 - 2*k12_2 - q2
    % Ans1 K22_1 =  -((2*k12_1 + q2)*((R1*R2*
    % (2*k12_2 + q2)^2)/(b^2*(2*R1*k12_2 + 2*R2*k12_1 + R1*q2 + R2*q2)))
    % ^(1/2))/(2*k12_2 + q2)
    
    % Ans2 K22_1 = ((2*k12_1 + q2)*((R1*R2*(2*k12_2 + q2)^2)
    % /(b^2*(2*R1*k12_2 + 2*R2*k12_1 + R1*q2 + R2*q2)))^(1/2))/(2*k12_2 + q2)
    
    % Ans1 K22_2 =  -((R1*R2*(2*k12_2 + q2)^2)/(b^2*
    % (2*R1*k12_2 + 2*R2*k12_1 + R1*q2 + R2*q2)))^(1/2)

    % Ans1 K22_2 = ((R1*R2*(2*k12_2 + q2)^2)/
    % (b^2*(2*R1*k12_2 + 2*R2*k12_1 + R1*q2 + R2*q2)))^(1/2)
    
    k22_1 = zeros(1, 2);
    k22_2 = zeros(1, 2);
    valid22 = [true; true]; % for validation in complex number
    if ((R1*R2*(2*k12_2(i) + q2)^2)/(b^2*(2*R1*k12_2(i) + 2*R2*k12_1(i) + R1*q2 + R2*q2))) < 0 
        valid22(i) = false;
    else
        k22_1(1) = -((2*k12_1(i) + q2)*((R1*R2*(2*k12_2(i) + q2)^2)/(b^2*(2*R1*k12_2(i) + 2*R2*k12_1(i) + R1*q2 + R2*q2)))^(1/2))/(2*k12_2(i) + q2);
    end
    if ((R1*R2*(2*k12_2(i) + q2)^2)/(b^2*(2*R1*k12_2(i) + 2*R2*k12_1(i) + R1*q2 + R2*q2))) < 0
        valid22(i) = false;
    else
        k22_1(2) =  ((2*k12_1(i) + q2)*((R1*R2*(2*k12_2(i) + q2)^2)/(b^2*(2*R1*k12_2(i) + 2*R2*k12_1(i) + R1*q2 + R2*q2)))^(1/2))/(2*k12_2(i) + q2);
    end
    if ((R1*R2*(2*k12_2(i) + q2)^2)/(b^2*(2*R1*k12_2(i) + 2*R2*k12_1(i) + R1*q2 + R2*q2))) < 0
        valid22(i) = false;
    else
        k22_2(1) = -((R1*R2*(2*k12_2(i) + q2)^2)/(b^2*(2*R1*k12_2(i) + 2*R2*k12_1(i) + R1*q2 + R2*q2)))^(1/2);
        k22_2(2) =  ((R1*R2*(2*k12_2(i) + q2)^2)/(b^2*(2*R1*k12_2(i) + 2*R2*k12_1(i) + R1*q2 + R2*q2)))^(1/2);
    end
    for j = 1:length(k22_1)
        if valid22(i) == false
            continue
        end
        % Last equation 
        % 1 (b^2*k12_1*k22_1)/R1 - a*k22_1 - k11_1 + (b^2*k12_2*k22_1)/R2
        % Ans k11_1 = (b^2*k12_1*k22_1)/R1 - a*k22_1 + (b^2*k12_2*k22_1)/R2
        % Ans k11_2 = (b^2*k12_1*k22_1)/R1 - a*k22_1 + (b^2*k12_2*k22_1)/R2
        k11_1 = (b^2*k12_1(i)*k22_1(j))/R1 - a*k22_1(j) + (b^2*k12_2(i)*k22_1(j))/R2;
        k11_2 = (b^2*k12_1(i)*k22_2(j))/R1 - a*k22_2(j) + (b^2*k12_2(i)*k22_2(j))/R2;
        temp_K_1 = zeros(2, 2);
        temp_K_1(1, 1) = k11_1;
        temp_K_1(1, 2) = k12_1(i);
        temp_K_1(2, 1) = k12_1(i);
        temp_K_1(2, 2) = k22_1(j);
        temp_K_2 = zeros(2, 2);
        temp_K_2(1, 1) = k11_2;
        temp_K_2(1, 2) = k12_2(i);
        temp_K_2(2, 1) = k12_2(i);
        temp_K_2(2, 2) = k22_2(j);
        if all(eig(A + (-B*R1_inv*B'*temp_K_1 - B*R2_inv*B'*temp_K_2)) < 0)
            k1_ans = temp_K_1;
            k2_ans = temp_K_2;
            valid_ans = true;
            break;
        end
        if valid_ans == true
            break;
        end
    end
    if valid_ans == true
        break;
    end
end

u2 = (R1_inv*B'*k1_ans) *pitch;

== matlab function Quad_Nonlinear_LQDG/SISO LQDG Controler/SISO LQDG/Roll LQDG Controller/Roll Function ==
  data: roll input; u1 output; q_roll input; q_p input; R_weight input; A1 input; A3 input
function u1 = fcn(roll, q_roll, q_p, R_weight, A1, A3)
% QuadConstants;
%%% constans %%%
% Distance between rotor center to quad center (m)
% d_cg = 0.295;
% Distance between D point to quad center (m)
% h_cg = 0.0078;
% Thrust factor (non dimensional)
% b = 1.10794e-5;
% Rotor torque drag factor (non dimensional)
% d = 3.2e-6;
% Total mass (kg)
% m_tot = 1.774;
% Quad Moment of inertia respect to axix X Body (kg.m^2)
% J_xx = 0.0297598;
% Quad Moment of inertia respect to axix Y Body (kg.m^2)
% J_yy = 0.0298565;
% Quad Moment of inertia respect to axix Y Body (kg.m^2)
% J_zz = 0.058510;
% Quad blade Moment (kg.m^2)
% J_R = 4.439e-5;
% Mass on X axis bearing (kg)
% m1 = 1.272;
% Mass on Y axis bearing (kg)
% m2 = 1.074;
% Mass on Z axis bearing (kg)
% m3 = 1.693;
% Bearing radius in X axix (m)
% r_x = 0.01;
% Bearing radius in Y axix (m)
% r_y = 0.01;
% Bearing radius in Z axix (m)
% r_z = 0.025;
% Static bearing friction (non dimensional)
% miu_s = 0.003;
% Dynamic bearing friction (non dimensional)
% miu_k = 0.002;
% Motor constant (non dimensional)
% tau = 0.15;
% Delay of motor (sec)
% T_d = 0.02;
% Gravity force (m/s^2)
% g = 9.81;
% A Constants
% A1 = (h_cg * g * m_tot) / (m_tot * h_cg^2 + J_xx);
% A2 = (2*m_tot * h_cg^2 + J_yy -J_zz) / (m_tot * h_cg^2 + J_xx);
% A3 = (b * d_cg) / (m_tot * h_cg^2 + J_xx);
% A4 = (J_R) / (m_tot * h_cg^2 + J_xx);
% A5 = (m1 * g * miu_k * r_x) / (m_tot * h_cg^2 + J_xx);
% B Constants
% B1 = (h_cg * g * m_tot) / (m_tot * h_cg^2 + J_yy);
% B2 = (-2*m_tot * h_cg^2 - J_xx + J_zz) / (m_tot * h_cg^2 + J_yy);
% B3 = (b * d_cg) / (m_tot * h_cg^2 + J_yy);
% B4 = (-J_R) / (m_tot * h_cg^2 + J_yy);
% B5 = (m2 * g * miu_k * r_y) / (m_tot * h_cg^2 + J_yy);
% C Constants
% C1 = (J_xx - J_yy) / (J_zz);
% C2 = (d) / (J_zz);
% C3 = (m3 * g * miu_k * r_z) / (J_zz);
% omega for linearzation 2000 RPM
% Omega = 2000 / 60 * 2 * pi;

x1     = roll(1);
A11    = 0; %da1dx1
A14    = 1; %da1dx4
A41    = A1 * cos(x1); %da4dx1
A44    = 0; %da4dx4

A      = [A11, A14 ;
          A41, A44];
B      = [0  ;
          A3];
a      = A(2);
b      = B(2);

q1     = 10^q_roll  ;
q2     = 10^q_p     ;
R1     = 1       ;
R2     = 10^R_weight;
R1_inv = R1^-1;
R2_inv = R2^-1;
k1_ans = zeros(2, 2);
k2_ans = zeros(2, 2);

% algebraic_riccati = K * A + A' * K - K * B * R^-1 * B' * K + Q;
% first equation q1 + 2*a*k12 - (b^2*k12^2)/R = 0
% Ans1 K12 = -m*(k + (k^2 + Q11)^(1/2))
% Ans2 K12 = -m*(k - (k^2 + Q11)^(1/2))
valid_ans = false; % answer validation for statble system
k12_1 = zeros(1, 2);
k12_2 = zeros(1, 2);
k12_1(1) =   (R1*R2*a + R1*b^2*((R1*R2*(R1*R2*a^2 + R1*b^2*q1 + R2*b^2*q1))/(b^4*(R1 + R2)^2))^(1/2) + R2*b^2*((R1*R2*(R1*R2*a^2 + R1*b^2*q1 + R2*b^2*q1))/(b^4*(R1 + R2)^2))^(1/2))/(R1*b^2 + R2*b^2);
k12_1(2) =  -(R1*b^2*((R1*R2*(R1*R2*a^2 + R1*b^2*q1 + R2*b^2*q1))/(b^4*(R1 + R2)^2))^(1/2) - R1*R2*a + R2*b^2*((R1*R2*(R1*R2*a^2 + R1*b^2*q1 + R2*b^2*q1))/(b^4*(R1 + R2)^2))^(1/2))/(R1*b^2 + R2*b^2);
k12_2(1) =  (R1*R2*a + R1*b^2*((R1*R2*(R1*R2*a^2 + R1*b^2*q1 + R2*b^2*q1))/(b^4*(R1 + R2)^2))^(1/2) + R2*b^2*((R1*R2*(R1*R2*a^2 + R1*b^2*q1 + R2*b^2*q1))/(b^4*(R1 + R2)^2))^(1/2))/(R1*b^2 + R2*b^2);
for i = 1:length(k12_1)
    % Second equation 
    % 1 (b^2*k22_1^2)/R1 + (k22_2*b^2*k22_1)/R2 - 2*k12_1 - q2 = 0
    % 2 (b^2*k22_2^2)/R2 + (k22_1*b^2*k22_2)/R1 - 2*k12_2 - q2
    % Ans1 K22_1 =  -((2*k12_1 + q2)*((R1*R2*
    % (2*k12_2 + q2)^2)/(b^2*(2*R1*k12_2 + 2*R2*k12_1 + R1*q2 + R2*q2)))
    % ^(1/2))/(2*k12_2 + q2)
    
    % Ans2 K22_1 = ((2*k12_1 + q2)*((R1*R2*(2*k12_2 + q2)^2)
    % /(b^2*(2*R1*k12_2 + 2*R2*k12_1 + R1*q2 + R2*q2)))^(1/2))/(2*k12_2 + q2)
    
    % Ans1 K22_2 =  -((R1*R2*(2*k12_2 + q2)^2)/(b^2*
    % (2*R1*k12_2 + 2*R2*k12_1 + R1*q2 + R2*q2)))^(1/2)

    % Ans1 K22_2 = ((R1*R2*(2*k12_2 + q2)^2)/
    % (b^2*(2*R1*k12_2 + 2*R2*k12_1 + R1*q2 + R2*q2)))^(1/2)
    
    k22_1 = zeros(1, 2);
    k22_2 = zeros(1, 2);
    valid22 = [true; true]; % for validation in complex number
    if ((R1*R2*(2*k12_2(i) + q2)^2)/(b^2*(2*R1*k12_2(i) + 2*R2*k12_1(i) + R1*q2 + R2*q2))) < 0 
        valid22(i) = false;
    else
        k22_1(1) = -((2*k12_1(i) + q2)*((R1*R2*(2*k12_2(i) + q2)^2)/(b^2*(2*R1*k12_2(i) + 2*R2*k12_1(i) + R1*q2 + R2*q2)))^(1/2))/(2*k12_2(i) + q2);
    end
    if ((R1*R2*(2*k12_2(i) + q2)^2)/(b^2*(2*R1*k12_2(i) + 2*R2*k12_1(i) + R1*q2 + R2*q2))) < 0
        valid22(i) = false;
    else
        k22_1(2) =  ((2*k12_1(i) + q2)*((R1*R2*(2*k12_2(i) + q2)^2)/(b^2*(2*R1*k12_2(i) + 2*R2*k12_1(i) + R1*q2 + R2*q2)))^(1/2))/(2*k12_2(i) + q2);
    end
    if ((R1*R2*(2*k12_2(i) + q2)^2)/(b^2*(2*R1*k12_2(i) + 2*R2*k12_1(i) + R1*q2 + R2*q2))) < 0
        valid22(i) = false;
    else
        k22_2(1) = -((R1*R2*(2*k12_2(i) + q2)^2)/(b^2*(2*R1*k12_2(i) + 2*R2*k12_1(i) + R1*q2 + R2*q2)))^(1/2);
        k22_2(2) =  ((R1*R2*(2*k12_2(i) + q2)^2)/(b^2*(2*R1*k12_2(i) + 2*R2*k12_1(i) + R1*q2 + R2*q2)))^(1/2);
    end
    for j = 1:length(k22_1)
        if valid22(i) == false
            continue
        end
        % Last equation 
        % 1 (b^2*k12_1*k22_1)/R1 - a*k22_1 - k11_1 + (b^2*k12_2*k22_1)/R2
        % Ans k11_1 = (b^2*k12_1*k22_1)/R1 - a*k22_1 + (b^2*k12_2*k22_1)/R2
        % Ans k11_2 = (b^2*k12_1*k22_1)/R1 - a*k22_1 + (b^2*k12_2*k22_1)/R2
        k11_1 = (b^2*k12_1(i)*k22_1(j))/R1 - a*k22_1(j) + (b^2*k12_2(i)*k22_1(j))/R2;
        k11_2 = (b^2*k12_1(i)*k22_2(j))/R1 - a*k22_2(j) + (b^2*k12_2(i)*k22_2(j))/R2;
        temp_K_1 = zeros(2, 2);
        temp_K_1(1, 1) = k11_1;
        temp_K_1(1, 2) = k12_1(i);
        temp_K_1(2, 1) = k12_1(i);
        temp_K_1(2, 2) = k22_1(j);
        temp_K_2 = zeros(2, 2);
        temp_K_2(1, 1) = k11_2;
        temp_K_2(1, 2) = k12_2(i);
        temp_K_2(2, 1) = k12_2(i);
        temp_K_2(2, 2) = k22_2(j);
        if all(eig(A + (-B*R1_inv*B'*temp_K_1 - B*R2_inv*B'*temp_K_2)) < 0)
            k1_ans = temp_K_1;
            k2_ans = temp_K_2;
            valid_ans = true;
            break;
        end
        if valid_ans == true
            break;
        end
    end
    if valid_ans == true
        break;
    end
end

u1 = (R1_inv*B'*k1_ans) *roll;

== matlab function Quad_Nonlinear_LQDG/SISO LQDG Controler/SISO LQDG/Yaw LQDG Controller/Yaw function ==
  data: yaw input; u3 output; q_yaw input; q_r input; R_weight input; C2 input
function u3 = fcn(yaw, q_yaw, q_r, R_weight, C2)
% QuadConstants;
%%% constans %%%
% Distance between rotor center to quad center (m)
% d_cg = 0.295;
% Distance between D point to quad center (m)
% h_cg = 0.0078;
% Thrust factor (non dimensional)
% b = 1.10794e-5;
% Rotor torque drag factor (non dimensional)
% d = 3.2e-6;
% Total mass (kg)
% m_tot = 1.774;
% Quad Moment of inertia respect to axix X Body (kg.m^2)
% J_xx = 0.0297598;
% Quad Moment of inertia respect to axix Y Body (kg.m^2)
% J_yy = 0.0298565;
% Quad Moment of inertia respect to axix Y Body (kg.m^2)
J_zz = 0.058510;
% Quad blade Moment (kg.m^2)
% J_R = 4.439e-5;
% Mass on X axis bearing (kg)
% m1 = 1.272;
% Mass on Y axis bearing (kg)
% m2 = 1.074;
% Mass on Z axis bearing (kg)
% m3 = 1.693;
% Bearing radius in X axix (m)
% r_x = 0.01;
% Bearing radius in Y axix (m)
% r_y = 0.01;
% Bearing radius in Z axix (m)
% r_z = 0.025;
% Static bearing friction (non dimensional)
% miu_s = 0.003;
% Dynamic bearing friction (non dimensional)
% miu_k = 0.002;
% Motor constant (non dimensional)
% tau = 0.15;
% Delay of motor (sec)
% T_d = 0.02;
% Gravity force (m/s^2)
% g = 9.81;
% A Constants
% A1 = (h_cg * g * m_tot) / (m_tot * h_cg^2 + J_xx);
% A2 = (2*m_tot * h_cg^2 + J_yy -J_zz) / (m_tot * h_cg^2 + J_xx);
% A3 = (b * d_cg) / (m_tot * h_cg^2 + J_xx);
% A4 = (J_R) / (m_tot * h_cg^2 + J_xx);
% A5 = (m1 * g * miu_k * r_x) / (m_tot * h_cg^2 + J_xx);
% B Constants
% B1 = (h_cg * g * m_tot) / (m_tot * h_cg^2 + J_yy);
% B2 = (-2*m_tot * h_cg^2 - J_xx + J_zz) / (m_tot * h_cg^2 + J_yy);
% B3 = (b * d_cg) / (m_tot * h_cg^2 + J_yy);
% B4 = (-J_R) / (m_tot * h_cg^2 + J_yy);
% B5 = (m2 * g * miu_k * r_y) / (m_tot * h_cg^2 + J_yy);
% C Constants
% C1 = (J_xx - J_yy) / (J_zz);
% C2 = (d) / (J_zz);
% C3 = (m3 * g * miu_k * r_z) / (J_zz);
% omega for linearzation 2000 RPM
% Omega = 2000 / 60 * 2 * pi;

A33    = 0; %da3dx3
A36    = 1; %da3dx6
A63    = 0; %da6dx3
A66    = 0; %da6dx6


A      = [A33, A36 ;
          A63, A66];
B      = [0  ;
          C2];
a      = A(2);
b      = B(2);

q1     = 10^q_yaw;
q2     = 10^q_r;
R1     = 1;
R2     = 10^R_weight;
R1_inv = R1^-1;
R2_inv = R2^-1;
k1_ans = zeros(2, 2);
k2_ans = zeros(2, 2);

% algebraic_riccati = K * A + A' * K - K * B * R^-1 * B' * K + Q;
% first equation q1 + 2*a*k12 - (b^2*k12^2)/R = 0
% Ans1 K12 = -m*(k + (k^2 + Q11)^(1/2))
% Ans2 K12 = -m*(k - (k^2 + Q11)^(1/2))
valid_ans = false; % answer validation for statble system
k12_1 = zeros(1, 2);
k12_2 = zeros(1, 2);
k12_1(1) =   (R1*R2*a + R1*b^2*((R1*R2*(R1*R2*a^2 + R1*b^2*q1 + R2*b^2*q1))/(b^4*(R1 + R2)^2))^(1/2) + R2*b^2*((R1*R2*(R1*R2*a^2 + R1*b^2*q1 + R2*b^2*q1))/(b^4*(R1 + R2)^2))^(1/2))/(R1*b^2 + R2*b^2);
k12_1(2) =  -(R1*b^2*((R1*R2*(R1*R2*a^2 + R1*b^2*q1 + R2*b^2*q1))/(b^4*(R1 + R2)^2))^(1/2) - R1*R2*a + R2*b^2*((R1*R2*(R1*R2*a^2 + R1*b^2*q1 + R2*b^2*q1))/(b^4*(R1 + R2)^2))^(1/2))/(R1*b^2 + R2*b^2);
k12_2(1) =  (R1*R2*a + R1*b^2*((R1*R2*(R1*R2*a^2 + R1*b^2*q1 + R2*b^2*q1))/(b^4*(R1 + R2)^2))^(1/2) + R2*b^2*((R1*R2*(R1*R2*a^2 + R1*b^2*q1 + R2*b^2*q1))/(b^4*(R1 + R2)^2))^(1/2))/(R1*b^2 + R2*b^2);
for i = 1:length(k12_1)
    % Second equation 
    % 1 (b^2*k22_1^2)/R1 + (k22_2*b^2*k22_1)/R2 - 2*k12_1 - q2 = 0
    % 2 (b^2*k22_2^2)/R2 + (k22_1*b^2*k22_2)/R1 - 2*k12_2 - q2
    % Ans1 K22_1 =  -((2*k12_1 + q2)*((R1*R2*
    % (2*k12_2 + q2)^2)/(b^2*(2*R1*k12_2 + 2*R2*k12_1 + R1*q2 + R2*q2)))
    % ^(1/2))/(2*k12_2 + q2)
    
    % Ans2 K22_1 = ((2*k12_1 + q2)*((R1*R2*(2*k12_2 + q2)^2)
    % /(b^2*(2*R1*k12_2 + 2*R2*k12_1 + R1*q2 + R2*q2)))^(1/2))/(2*k12_2 + q2)
    
    % Ans1 K22_2 =  -((R1*R2*(2*k12_2 + q2)^2)/(b^2*
    % (2*R1*k12_2 + 2*R2*k12_1 + R1*q2 + R2*q2)))^(1/2)

    % Ans1 K22_2 = ((R1*R2*(2*k12_2 + q2)^2)/
    % (b^2*(2*R1*k12_2 + 2*R2*k12_1 + R1*q2 + R2*q2)))^(1/2)
    
    k22_1 = zeros(1, 2);
    k22_2 = zeros(1, 2);
    valid22 = [true; true]; % for validation in complex number
    if ((R1*R2*(2*k12_2(i) + q2)^2)/(b^2*(2*R1*k12_2(i) + 2*R2*k12_1(i) + R1*q2 + R2*q2))) < 0 
        valid22(i) = false;
    else
        k22_1(1) = -((2*k12_1(i) + q2)*((R1*R2*(2*k12_2(i) + q2)^2)/(b^2*(2*R1*k12_2(i) + 2*R2*k12_1(i) + R1*q2 + R2*q2)))^(1/2))/(2*k12_2(i) + q2);
    end
    if ((R1*R2*(2*k12_2(i) + q2)^2)/(b^2*(2*R1*k12_2(i) + 2*R2*k12_1(i) + R1*q2 + R2*q2))) < 0
        valid22(i) = false;
    else
        k22_1(2) =  ((2*k12_1(i) + q2)*((R1*R2*(2*k12_2(i) + q2)^2)/(b^2*(2*R1*k12_2(i) + 2*R2*k12_1(i) + R1*q2 + R2*q2)))^(1/2))/(2*k12_2(i) + q2);
    end
    if ((R1*R2*(2*k12_2(i) + q2)^2)/(b^2*(2*R1*k12_2(i) + 2*R2*k12_1(i) + R1*q2 + R2*q2))) < 0
        valid22(i) = false;
    else
        k22_2(1) = -((R1*R2*(2*k12_2(i) + q2)^2)/(b^2*(2*R1*k12_2(i) + 2*R2*k12_1(i) + R1*q2 + R2*q2)))^(1/2);
        k22_2(2) =  ((R1*R2*(2*k12_2(i) + q2)^2)/(b^2*(2*R1*k12_2(i) + 2*R2*k12_1(i) + R1*q2 + R2*q2)))^(1/2);
    end
    for j = 1:length(k22_1)
        if valid22(i) == false
            continue
        end
        % Last equation 
        % 1 (b^2*k12_1*k22_1)/R1 - a*k22_1 - k11_1 + (b^2*k12_2*k22_1)/R2
        % Ans k11_1 = (b^2*k12_1*k22_1)/R1 - a*k22_1 + (b^2*k12_2*k22_1)/R2
        % Ans k11_2 = (b^2*k12_1*k22_1)/R1 - a*k22_1 + (b^2*k12_2*k22_1)/R2
        k11_1 = (b^2*k12_1(i)*k22_1(j))/R1 - a*k22_1(j) + (b^2*k12_2(i)*k22_1(j))/R2;
        k11_2 = (b^2*k12_1(i)*k22_2(j))/R1 - a*k22_2(j) + (b^2*k12_2(i)*k22_2(j))/R2;
        temp_K_1 = zeros(2, 2);
        temp_K_1(1, 1) = k11_1;
        temp_K_1(1, 2) = k12_1(i);
        temp_K_1(2, 1) = k12_1(i);
        temp_K_1(2, 2) = k22_1(j);
        temp_K_2 = zeros(2, 2);
        temp_K_2(1, 1) = k11_2;
        temp_K_2(1, 2) = k12_2(i);
        temp_K_2(2, 1) = k12_2(i);
        temp_K_2(2, 2) = k22_2(j);
        if all(eig(A + (-B*R1_inv*B'*temp_K_1 - B*R2_inv*B'*temp_K_2)) < 0)
            k1_ans = temp_K_1;
            k2_ans = temp_K_2;
            valid_ans = true;
            break;
        end
        if valid_ans == true
            break;
        end
    end
    if valid_ans == true
        break;
    end
end

u3 = (R1_inv*B'*k1_ans + R2_inv*B'*k2_ans) *yaw;
